simulink library "VsrLibDriveCycleSrc"  (R2019b)
settings: Solver=VariableStepAuto  StartTime=0.0  StopTime=10.0  RelTol=1e-3
undefined symbols (not defined in the file): objs, PtbsDriveCycleStructArray, TimeLookAhead
libraries: simulink x2, $bdroot x1
settings Model: Creator=9bt  LastModifiedBy=4qz

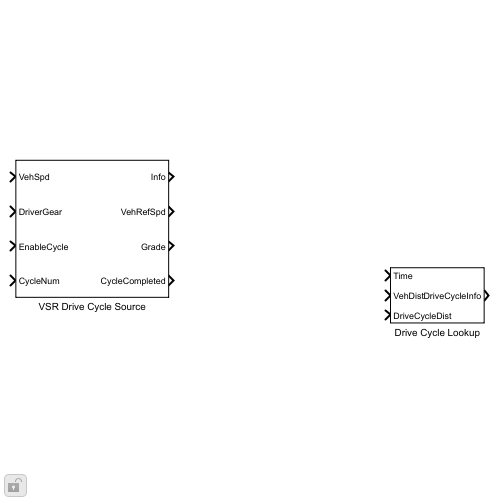
[thumbnail: Simulink's stored preview of the top-level diagram]
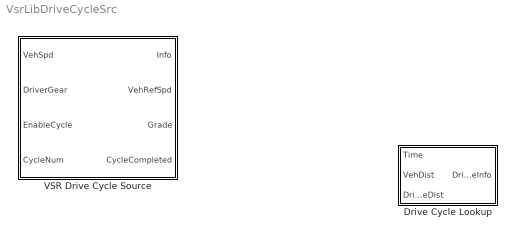
== system VsrLibDriveCycleSrc ==
  Drive Cycle Lookup : Subsystem  mask{DriveCycleStruct=objs(1).getCycleDataStruct, TimeLookAhead=TimeLookAhead}
      mask prompts: DriveCycleStruct "Drive cycle struct"; TimeLookAhead "Look ahead time, TimeLookAhead [s]:"
      mask init:
      | obj = vsr.mdl.drivecycle.DriveCycleLookupBlkCtrl(gcb);
      | MaskData = obj.Init;
  VSR Drive Cycle Source : Subsystem  mask{DistCompensationCheckbox=off, DriveCycleStructArray=PtbsDriveCycleStructArray(1:30), TimeLookAhead=0.5}
      mask prompts: DistCompensationCheckbox "Use distance compensation"; DriveCycleStructArray "Array of drive cycle structs, DriveCycleStructArray (vsr.drivecycle.DriveCycle.getCycleDataStruct)"; TimeLookAhead "Look ahead time, TimeLookAhead [s]:"
      mask init:
      | obj = vsr.mdl.drivecycle.DriveCycleSrcBlkCtrl(gcb);
      | MaskData = obj.Init;

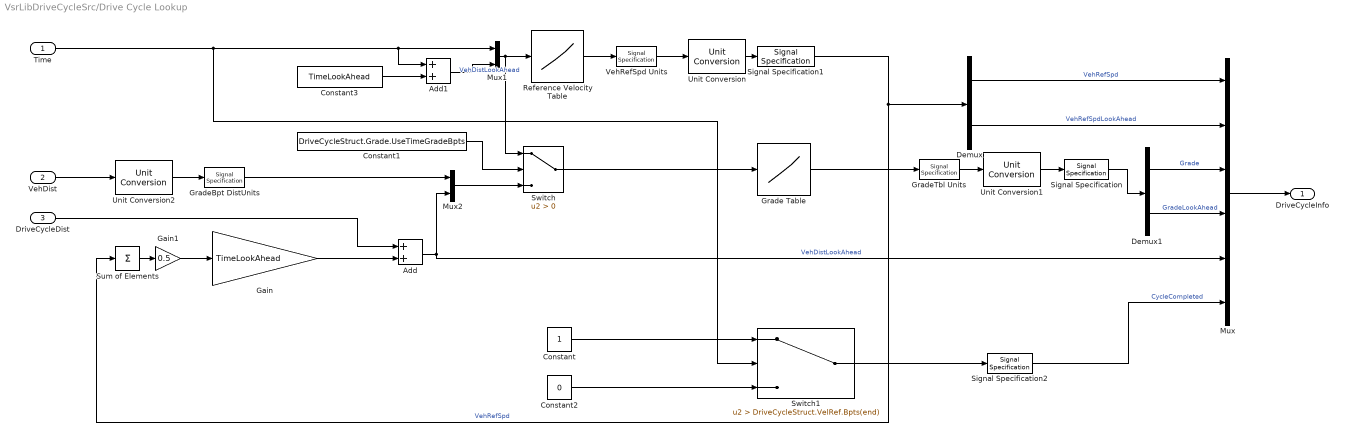
== system VsrLibDriveCycleSrc/Drive Cycle Lookup ==
  Time : Inport
  VehDist : Inport  Port=2  Unit=m
  DriveCycleDist : Inport  Port=3  Unit=m
  Add : Sum
  Add1 : Sum
  Constant : Constant
  Constant1 : Constant  Value=DriveCycleStruct.Grade.UseTimeGradeBpts
  Constant2 : Constant  Value=0
  Constant3 : Constant  Value=TimeLookAhead  SampleTime=-1
  Demux : Demux  Outputs=2
  Demux1 : Demux  Outputs=2
  Gain : Gain  Gain=TimeLookAhead
  Gain1 : Gain  Gain=0.5
  Grade Table : Lookup_n-D  NumberOfTableDimensions=1  LookupTableObject=''  BreakpointsForDimension1=DriveCycleStruct.Grade.Bpts  BeginIndexSearchUsingPreviousIndexResult=on  Table=DriveCycleStruct.Grade.Tbl  ExtrapMethod=Clip  RemoveProtectionInput=on  UseLastTableValue=on  InternalRulePriority=Speed  RndMeth=Simplest  InputSameDT=on
  GradeBpt DistUnits : SignalSpecification  Unit=m
  GradeTbl Units : SignalSpecification  Unit=rad
  Mux : Mux  Inputs=6
  Mux1 : Mux  Inputs=2
  Mux2 : Mux  Inputs=2
  Reference Velocity Table : Lookup_n-D  NumberOfTableDimensions=1  LookupTableObject=''  BreakpointsForDimension1=DriveCycleStruct.VelRef.Bpts  BeginIndexSearchUsingPreviousIndexResult=on  Table=DriveCycleStruct.VelRef.Tbl  ExtrapMethod=Clip  RemoveProtectionInput=on  UseLastTableValue=on  InternalRulePriority=Speed  RndMeth=Simplest  InputSameDT=on
  Signal Specification : SignalSpecification  Unit=rad
  Signal Specification1 : SignalSpecification  Unit=m/s
  Signal Specification2 : SignalSpecification  OutDataTypeStr=double
  Sum of Elements : Sum  Inputs=+
  Switch : Switch  Criteria=u2 > Threshold  ZeroCross=off
  Switch1 : Switch  Criteria=u2 > Threshold  Threshold=DriveCycleStruct.VelRef.Bpts(end)  ZeroCross=off
  Unit Conversion : UnitConversion
  Unit Conversion1 : UnitConversion
  Unit Conversion2 : UnitConversion
  VehRefSpd Units : SignalSpecification  Unit=m/s
  DriveCycleInfo : Outport
  wires:
  Reference Velocity Table/1 -> VehRefSpd Units/1
  Grade Table/1 -> GradeTbl Units/1
  Mux/1 -> DriveCycleInfo/1
  VehDist/1 -> Unit Conversion2/1
  Time/1 -> Add1/1, Mux1/1, Switch1/2
  Demux1/1 -> Mux/3  "Grade"
  Switch/1 -> Grade Table/1
  Demux/1 -> Mux/1  "VehRefSpd"
  VehRefSpd Units/1 -> Unit Conversion/1
  Unit Conversion/1 -> Signal Specification1/1
  Constant1/1 -> Switch/2
  Signal Specification2/1 -> Mux/6  "CycleCompleted"
  Switch1/1 -> Signal Specification2/1
  Constant/1 -> Switch1/1
  Constant2/1 -> Switch1/3
  Unit Conversion1/1 -> Signal Specification/1
  GradeTbl Units/1 -> Unit Conversion1/1
  GradeBpt DistUnits/1 -> Mux2/1
  Unit Conversion2/1 -> GradeBpt DistUnits/1
  Constant3/1 -> Add1/2
  Mux1/1 -> Switch/1, Reference Velocity Table/1
  Signal Specification1/1 -> Sum of Elements/1, Demux/1  "VehRefSpd"
  Demux/2 -> Mux/2  "VehRefSpdLookAhead"
  Mux2/1 -> Switch/3
  Signal Specification/1 -> Demux1/1
  Demux1/2 -> Mux/4  "GradeLookAhead"
  Add/1 -> Mux/5, Mux2/2  "VehDistLookAhead"
  Gain/1 -> Add/2
  Gain1/1 -> Gain/1
  Sum of Elements/1 -> Gain1/1
  Add1/1 -> Mux1/2  "VehDistLookAhead"
  DriveCycleDist/1 -> Add/1

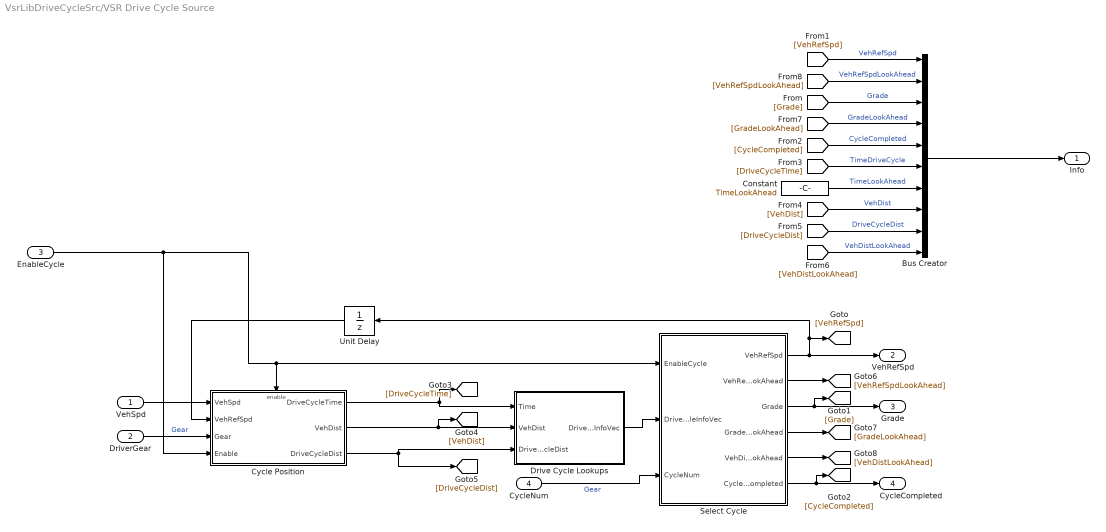
== system VsrLibDriveCycleSrc/VSR Drive Cycle Source ==
  VehSpd : Inport
  DriverGear : Inport  Port=2
  EnableCycle : Inport  Port=3
  CycleNum : Inport  Port=4
  Bus Creator : BusCreator  Inputs=10
  Constant : Constant  Value=TimeLookAhead
  Cycle Position : Subsystem
  Drive Cycle Lookups : Subsystem
  Select Cycle : Subsystem
  Unit Delay : UnitDelay  SampleTime=-1  HasFrameUpgradeWarning=on
  Info : Outport
  VehRefSpd : Outport  Port=2  Unit=m/s
  Grade : Outport  Port=3  Unit=rad
  CycleCompleted : Outport  Port=4
  wires:
  Unit Delay/1 -> Cycle Position/2(VehRefSpd)
  VehSpd/1 -> Cycle Position/1(VehSpd)
  Select Cycle/1(VehRefSpd) -> VehRefSpd/1, Unit Delay/1, [VehRefSpd]
  DriverGear/1 -> Cycle Position/3(Gear)  "Gear"
  Cycle Position/1(DriveCycleTime) -> Drive Cycle Lookups/1(Time), [DriveCycleTime]
  EnableCycle/1 -> Cycle Position/Enable, Select Cycle/1(EnableCycle), Cycle Position/4(Enable)
  Drive Cycle Lookups/1(DriveCycleInfoVec) -> Select Cycle/2(DriveCycleInfoVec)
  CycleNum/1 -> Select Cycle/3(CycleNum)  "Gear"
  Select Cycle/3(Grade) -> [Grade], Grade/1
  Select Cycle/6(CycleCompleted) -> [CycleCompleted], CycleCompleted/1
  Bus Creator/1 -> Info/1
  [VehRefSpd] -> Bus Creator/1  "VehRefSpd"
  [Grade] -> Bus Creator/3  "Grade"
  [CycleCompleted] -> Bus Creator/5  "CycleCompleted"
  [DriveCycleTime] -> Bus Creator/6  "TimeDriveCycle"
  Cycle Position/2(VehDist) -> Drive Cycle Lookups/2(VehDist), [VehDist]
  Cycle Position/3(DriveCycleDist) -> [DriveCycleDist], Drive Cycle Lookups/3(DriveCycleDist)
  [VehDist] -> Bus Creator/8  "VehDist"
  [DriveCycleDist] -> Bus Creator/9  "DriveCycleDist"
  Select Cycle/2(VehRefSpdLookAhead) -> [VehRefSpdLookAhead]
  Select Cycle/4(GradeLookAhead) -> [GradeLookAhead]
  Select Cycle/5(VehDistLookAhead) -> [VehDistLookAhead]
  [VehDistLookAhead] -> Bus Creator/10  "VehDistLookAhead"
  [GradeLookAhead] -> Bus Creator/4  "GradeLookAhead"
  [VehRefSpdLookAhead] -> Bus Creator/2  "VehRefSpdLookAhead"
  Constant/1 -> Bus Creator/7  "TimeLookAhead"

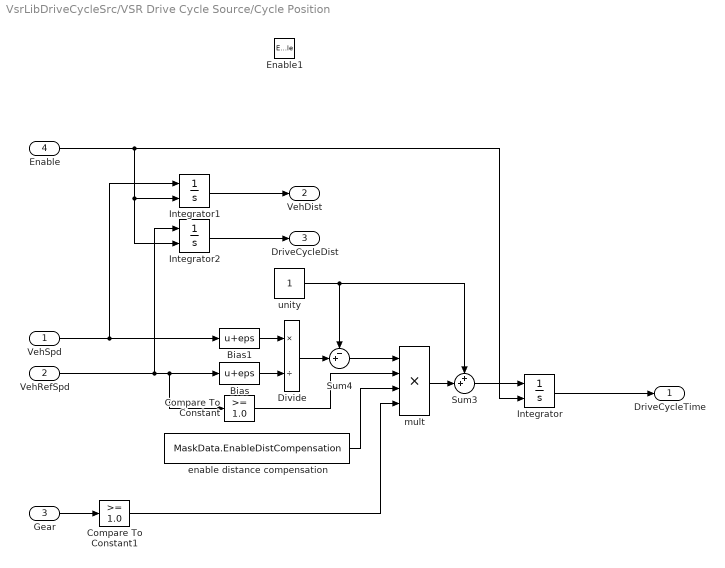
== system VsrLibDriveCycleSrc/VSR Drive Cycle Source/Cycle Position ==
  VehSpd : Inport
  VehRefSpd : Inport  Port=2
  Gear : Inport  Port=3
  Enable : Inport  Port=4
  Enable1 : EnablePort  StatesWhenEnabling=reset
  Bias : Bias  Bias=eps
  Bias1 : Bias  Bias=eps
  Compare To Constant : simulink/Logic and Bit Operations/Compare To Constant  relop=>=  const=1.0  OutDataTypeStr=boolean  ZeroCross=off
  Compare To Constant1 : simulink/Logic and Bit Operations/Compare To Constant  relop=>=  const=1.0  OutDataTypeStr=boolean  ZeroCross=off
  Divide : Product  Inputs=*/
  Integrator : Integrator  ExternalReset=rising  ZeroCross=off
  Integrator1 : Integrator  ExternalReset=rising  ZeroCross=off
  Integrator2 : Integrator  ExternalReset=rising  ZeroCross=off
  Sum3 : Sum  Inputs=++|
  Sum4 : Sum  Inputs=-+|
  enable distance compensation : Constant  Value=MaskData.EnableDistCompensation
  mult : Product  Inputs=4
  unity : Constant
  DriveCycleTime : Outport  PortDimensions=1
  VehDist : Outport  Port=2  Unit=m  LockScale=on
  DriveCycleDist : Outport  Port=3  Unit=m
  wires:
  Enable/1 -> Integrator/2, Integrator1/2, Integrator2/2
  Compare To Constant1/1 -> mult/4
  mult/1 -> Sum3/2
  enable distance compensation/1 -> mult/3
  VehSpd/1 -> Integrator1/1, Bias1/1
  Sum4/1 -> mult/1
  Compare To Constant/1 -> mult/2
  unity/1 -> Sum3/1, Sum4/1
  Divide/1 -> Sum4/2
  Sum3/1 -> Integrator/1
  Bias/1 -> Divide/2
  Bias1/1 -> Divide/1
  Gear/1 -> Compare To Constant1/1
  VehRefSpd/1 -> Integrator2/1, Bias/1, Compare To Constant/1
  Integrator1/1 -> VehDist/1
  Integrator2/1 -> DriveCycleDist/1
  Integrator/1 -> DriveCycleTime/1

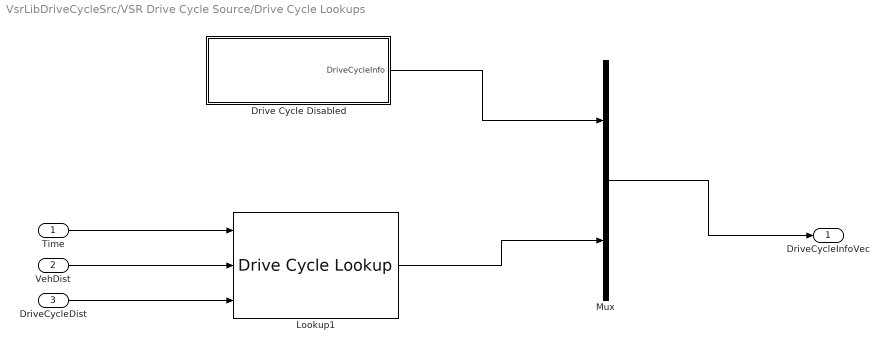
== system VsrLibDriveCycleSrc/VSR Drive Cycle Source/Drive Cycle Lookups ==
  Time : Inport
  VehDist : Inport  Port=2
  DriveCycleDist : Inport  Port=3
  Drive Cycle Disabled : Subsystem
  Lookup1 : $bdroot/Drive Cycle Lookup  DriveCycleStruct=MaskData.DriveCycleData1  TimeLookAhead=TimeLookAhead
  Mux : Mux  Inputs=2
  DriveCycleInfoVec : Outport
  wires:
  Mux/1 -> DriveCycleInfoVec/1
  Drive Cycle Disabled/1(DriveCycleInfo) -> Mux/1
  Time/1 -> Lookup1/1
  VehDist/1 -> Lookup1/2
  Lookup1/1 -> Mux/2
  DriveCycleDist/1 -> Lookup1/3

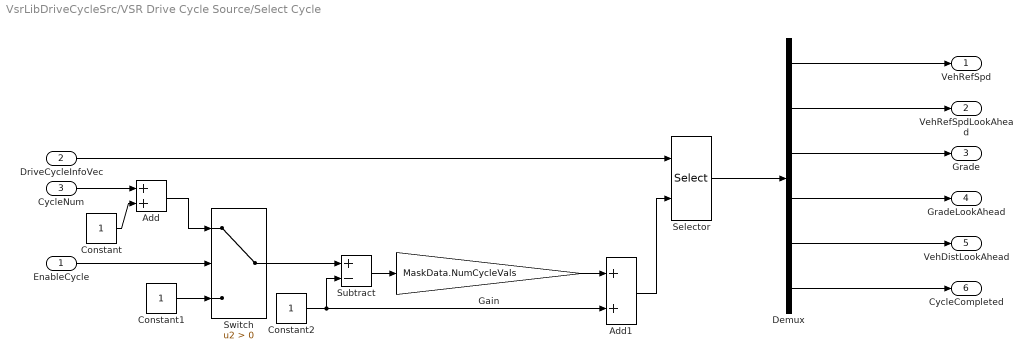
== system VsrLibDriveCycleSrc/VSR Drive Cycle Source/Select Cycle ==
  EnableCycle : Inport
  DriveCycleInfoVec : Inport  Port=2
  CycleNum : Inport  Port=3
  Add : Sum
  Add1 : Sum
  Constant : Constant
  Constant1 : Constant
  Constant2 : Constant
  Demux : Demux  Outputs=6
  Gain : Gain  Gain=MaskData.NumCycleVals
  Selector : Selector  InputPortWidth=(MaskData.NumCycles+1)*MaskData.NumCycleVals  IndexOptions=Starting index (port)  Indices=[1 3]  OutputSizes=6
  Subtract : Sum  Inputs=+-
  Switch : Switch  Criteria=u2 > Threshold
  VehRefSpd : Outport
  VehRefSpdLookAhead : Outport  Port=2
  Grade : Outport  Port=3
  GradeLookAhead : Outport  Port=4
  VehDistLookAhead : Outport  Port=5
  CycleCompleted : Outport  Port=6
  wires:
  Selector/1 -> Demux/1
  DriveCycleInfoVec/1 -> Selector/1
  CycleNum/1 -> Add/1
  Demux/1 -> VehRefSpd/1
  Demux/3 -> Grade/1
  Demux/6 -> CycleCompleted/1
  Constant/1 -> Add/2
  EnableCycle/1 -> Switch/2
  Add/1 -> Switch/1
  Constant1/1 -> Switch/3
  Switch/1 -> Subtract/1
  Constant2/1 -> Subtract/2, Add1/2
  Subtract/1 -> Gain/1
  Add1/1 -> Selector/2
  Gain/1 -> Add1/1
  Demux/2 -> VehRefSpdLookAhead/1
  Demux/4 -> GradeLookAhead/1
  Demux/5 -> VehDistLookAhead/1

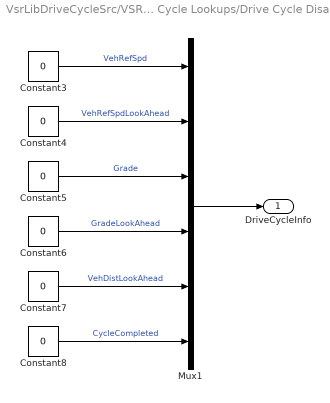
== system VsrLibDriveCycleSrc/VSR Drive Cycle Source/Drive Cycle Lookups/Drive Cycle Disabled ==
  Constant{3..8} (6 alike) : Constant  Value=0
  Mux1 : Mux  Inputs=6
  DriveCycleInfo : Outport
  wires:
  Mux1/1 -> DriveCycleInfo/1
  Constant5/1 -> Mux1/3  "Grade"
  Constant6/1 -> Mux1/4  "GradeLookAhead"
  Constant8/1 -> Mux1/6  "CycleCompleted"
  Constant7/1 -> Mux1/5  "VehDistLookAhead"
  Constant4/1 -> Mux1/2  "VehRefSpdLookAhead"
  Constant3/1 -> Mux1/1  "VehRefSpd"
